simulink library "uavsimblockset_PilotCommands"  (Simulink 8.0)
settings: Solver=ode45  StartTime=0.0  StopTime=10.0  RelTol=1e-3
libraries: aerolibanimutils x1
settings Model: Creator=mstolle  LastModifiedBy=j.bolting

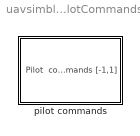
== system uavsimblockset_PilotCommands ==
  pilot commands : Subsystem

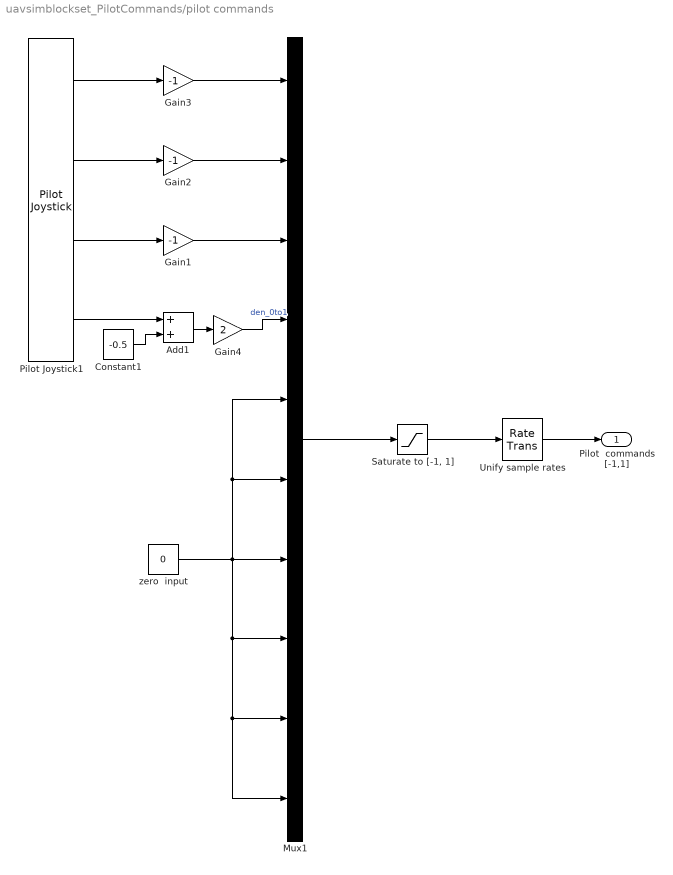
== system uavsimblockset_PilotCommands/pilot commands ==
  Add1 : Sum
  Constant1 : Constant  Value=-0.5
  Gain1 : Gain  Gain=-1
  Gain2 : Gain  Gain=-1
  Gain3 : Gain  Gain=-1
  Gain4 : Gain  Gain=2
  Mux1 : Mux  Inputs=10
  Pilot Joystick1 : aerolibanimutils/Pilot Joystick  JoystickID=Joystick1  OutputConfiguration=FourAxis  SampleTime=1/10
  "Saturate to [-1, 1]" : Saturate  UpperLimit=1  LowerLimit=-1
  Unify sample rates : RateTransition
  zero  input : Constant  Value=0
  Pilot  commands [-1,1] : Outport
  wires:
  Pilot Joystick1/1 -> Gain3/1
  Pilot Joystick1/2 -> Gain2/1
  Pilot Joystick1/3 -> Gain1/1
  Mux1/1 -> "Saturate to [-1, 1]"/1
  zero  input/1 -> Mux1/10, Mux1/9, Mux1/8, Mux1/7, Mux1/6, Mux1/5
  Unify sample rates/1 -> Pilot  commands [-1,1]/1
  Add1/1 -> Gain4/1
  Constant1/1 -> Add1/2
  Pilot Joystick1/4 -> Add1/1
  Gain4/1 -> Mux1/4  "den_0to1"
  "Saturate to [-1, 1]"/1 -> Unify sample rates/1
  Gain1/1 -> Mux1/3
  Gain2/1 -> Mux1/2
  Gain3/1 -> Mux1/1
